simulink model "sm_boom_lift_crawler_test_basket_level_tilt_hydr"  (R2026a)
settings: Solver=ode23t  StopTime=tVec.StopTime  AbsTol=1e-3
PostLoadFcn:
  | sm_boom_lift_crawler_settest('tilt test')
StartFcn:
  | tic;
StopFcn:
  | Elapsed_Sim_Time = toc;
  | %disp(['Elapsed Sim Time = ' num2str(Elapsed_Sim_Time)]);
undefined symbols (not defined in the file): oVec, tVec, X, Y, Z
libraries: sm_boom_lift_crawler_lib x8, nesl_utility x5, sm_lib x3, sm_boom_lift_crawler_lib_actuators x2, sm_boom_lift_crawler_lib_boom x2, fl_lib x2, sm_boom_lift_crawler_lib_inputs x1
Description:
  | Copyright 2025-2026 The MathWorks, Inc.
settings Model: Creator=smiller  LastModifiedBy=smiller
settings SolverCC: MaxConsecutiveMinStep=3
settings DataIOCC: SignalLoggingName=logsout_sm_boom_lift_crawler
settings SimscapeCC: SimscapeNominalValues="[{\"value\":\"1\",\"unit\":\"A\"},{\"value\":\"nomval_psi\",\"unit\":\"psi\"},{\"value\":\"1\",\"unit\":\"cm^2\"},{\"value\":\"nomval_cmv3_s\",\"unit\":\"cm^3/s\"},{\"value\":\"1\",\"unit\":\"kJ/kg\"},{\"value\":\"1\",\"unit\":\"kW\"},{\"value\":\"1\",\"unit\":\"l\"},{\"value\":\"nomval_N\",\"unit\":\"N\"},{\"value\":\"nomval_Nm\",\"unit\":\"N*m\"},{\"value\":\"1\",\"unit\":\"V\"}]"  SimscapeLogName=simlog_sm_boom_lift_crawler  SimscapeLogLimitData=off  SimscapeLogDataHistory=5000.0
settings DiagnosticsConfigSet: SimMechanicsConflictingReferenceFrames=none  SimMechanicsRigidlyBoundBlock=none
settings ExplorerConfigSet: InternalSimMechanicsExplorerSettings="<ExplorerConfiguration><canonicalview>default</canonicalview><AnimationSetting><BasePlaybackSpeed>1.0</BasePlaybackSpeed><PlaybackSpeedFactor>8.0</PlaybackSpeedFactor></AnimationSetting><TilePanel><TileInfo><Tiles Columns=\"1\" Count=\"1\" Rows=\"1\"><Column Weight=\"1\"/><Row Weight=\"1\"/><Tile Height=\"1\" Width=\"1\" X=\"0\" Y=\"0\"/></Tiles></TileInfo><SceneInfo><SceneViewer><BGColor><R>1</R><G>1</G><B>1</B></BGColor><Camera><DoPerspective>on</DoPerspective><Position><X>-2.99999999999999512</X><Y>3.60557049947193109</Y><Z>1.13505049508107825</Z></Position><Center><X>-1.99999999999999512</X><Y>3.60557049947193109</Y><Z>1.13505049508107803</Z></Center><Up><X>0</X><Y>0</Y><Z>1</Z></Up><ViewLimDist>1</ViewLimDist><YLim>0.466307658154998583</YLim><XLim>0.327096812401001136</XLim></Camera></SceneViewer></SceneInfo></TilePanel><MechEditorPanel><Cameras><Camera><Id>Camera8</Id><Value><Name>Extend_Knuckle</Name><NativeCamera><PositionTrackingFeature>Boom.Arms.Telescope.Extend_Cylinder.Transform_Camera_Extend_Knuckle.F</PositionTrackingFeature><CenterTrackingFeature>Boom.Arms.Telescope.Extend_Cylinder.Transform_Camera_Extend_Knuckle.F</CenterTrackingFeature><UpVectorTrackingFeature>Boom.Arms.Telescope.Extend_Cylinder.Transform_Camera_Extend_Knuckle.F</UpVectorTrackingFeature><CenterTrackingOrigin>off</CenterTrackingOrigin><CenterTrackingDirection>-X</CenterTrackingDirection><UpVectorTrackingDirection>-Y</UpVectorTrackingDirection></NativeCamera></Value></Camera><Camera><Id>Camera9</Id><Value><Name>Extend_Basket</Name><NativeCamera><PositionTrackingFeature>Boom.Arms.Telescope.Extend_Cylinder.Transform_Camera_Extend_Basket.F</PositionTrackingFeature><CenterTrackingFeature>Boom.Arms.Telescope.Extend_Cylinder.Transform_Camera_Extend_Basket.F</CenterTrackingFeature><UpVectorTrackingFeature>Boom.Arms.Telescope.Extend_Cylinder.Transform_Camera_Extend_Basket.F</UpVectorTrackingFeature><CenterTrackingOrigin>off</CenterTrackingOrigin><CenterTrackingDirection>+X</CenterTrackingDirection><UpVectorTrackingDirection>+Y</UpVectorTrackingDirection></NativeCamera></Value></Camera><Camera><Id>Camera10</Id><Value><Name>Basket_Rotate</Name><NativeCamera><PositionTrackingFeature>Boom.Basket.Basket_Rotate.Bracket.Reference_Camera_Basket_Rotate_L.R</PositionTrackingFeature><CenterTrackingFeature>Boom.Basket.Basket_Rotate.Bracket.Reference_Camera_Basket_Rotate_L.R</CenterTrackingFeature><UpVectorTrackingFeature>Boom.Basket.Basket_Rotate.Bracket.Reference_Camera_Basket_Rotate_L.R</UpVectorTrackingFeature><CenterTrackingOrigin>off</CenterTrackingOrigin><CenterTrackingDirection>-X</CenterTrackingDirection><UpVectorTrackingDirection>+Z</UpVectorTrackingDirection></NativeCamera></Value></Camera><Camera><Id>Camera11</Id><Value><Name>Tilt_Knuckle</Name><NativeCamera><PositionTrackingFeature>Boom.Arms.Tower.Upper_Knuckle.Reference_Knuckle_Cam.R</PositionTrackingFeature><CenterTrackingFeature>Boom.Arms.Tower.Upper_Knuckle.Reference_Knuckle_Cam.R</CenterTrackingFeature><UpVectorTrackingFeature>Mech_Config.World.W</UpVectorTrackingFeature><CenterTrackingOrigin>off</CenterTrackingOrigin><CenterTrackingDirection>+Z</CenterTrackingDirection><UpVectorTrackingDirection>+Z</UpVectorTrackingDirection></NativeCamera></Value></Camera><Camera><Id>Camera12</Id><Value><Name>Full Test</Name><NativeCamera><PositionKeyframeSet><Keyframe><Time>0</Time><Value><X>-12.242458171438994</X><Y>-0.1433452642095574</Y><Z>4.1505972342390427</Z></Value></Keyframe><Keyframe><Time>69.026826430124729</Time><Value><X>-14.974593328379619</X><Y>0.0056652615564253064</Y><Z>5.3389029552684786</Z></Value></Keyframe><Keyframe><Time>110.29539843687829</Time><Value><X>-21.00761369699504</X><Y>-0.0057417156870510078</Y><Z>8.0689402037867488</Z></Value></Keyframe><Keyframe><Time>140.70430157635164</Time><Value><X>-31.272784439198116</X><Y>-2.5583130214499052e-10</Y><Z>12.723321478963756</Z></Value></Keyframe><Keyframe><Time>181.77628976806102</Time><Value><X>-31.272784439198116</X><Y>-2.5583130214499052e-10</Y><Z>12.723321478963756</Z></Value></Keyframe><Keyframe><Time>208.0087867386398</Time><Value><X>-23.351505250921551</X><Y>-2.5583182919801497e-10</Y><Z>9.1371534281977738</Z></Value></Keyframe><Keyframe><Time>243.06358572448306</Time><Value><X>-16.577121762622586</X><Y>-2.5583144573665537e-10</Y><Z>6.0702143126734844</Z></Value></Keyframe><Keyframe><Time>273.3415757110605</Time><Value><X>-16.577121762622586</X><Y>-2.5583144573665537e-10</Y><Z>6.0702143126734844</Z></Value></Keyframe><Keyframe><Time>321.2447002217541</Time><Value><X>-13.690590902490033</X><Y>0.01787769923724114</Y><Z>4.7891626503614262</Z></Value></Keyframe><Keyframe><Time>350</Time><Value><X>-13.690590902490033</X><Y>0.01787769923724114</Y><Z>4.7891626503614262</Z></Value></Keyframe></PositionKeyframeSet><CenterKeyframeSet><Keyframe><Time>0</Time><Value><X>-4.621228999686064</X><Y>-0.1433452642095574</Y><Z>4.1505972342390436</Z></Value></Keyframe><Keyframe><Time>69.026826430124729</Time><Value><X>-0.17395018713353672</X><Y>0.0056652615564253064</Y><Z>5.3389029552684786</Z></Value></Keyframe><Keyframe><Time>110.29539843687829</Time><Value><X>-9.0038066291239502</X><Y>-0.0057417156870549491</Y><Z>8.0689402037867524</Z></Value></Keyframe><Keyframe><Time>140.70430157635164</Time><Value><X>-14.136391845814327</X><Y>-2.5583979379462107e-10</Y><Z>12.72332147896376</Z></Value></Keyframe><Keyframe><Time>181.77628976806102</Time><Value><X>-2.3429975002054775</X><Y>-2.5584563781180217e-10</Y><Z>12.723321478963761</Z></Value></Keyframe><Keyframe><Time>208.0087867386398</Time><Value><X>-10.17575261115104</X><Y>-2.5583801743778167e-10</Y><Z>9.1371534281977755</Z></Value></Keyframe><Keyframe><Time>243.06358572448306</Time><Value><X>-0.54476849060194255</X><Y>-2.5583897563257738e-10</Y><Z>6.0702143126734844</Z></Value></Keyframe><Keyframe><Time>273.3415757110605</Time><Value><X>-0.11057247639663359</X><Y>-2.5583917956089291e-10</Y><Z>6.0702143126734844</Z></Value></Keyframe><Keyframe><Time>321.2447002217541</Time><Value><X>-5.3452949964231387</X><Y>0.017877699237237366</Y><Z>4.7891626503614253</Z></Value></Keyframe><Keyframe><Time>350</Time><Value><X>-5.3452949964231387</X><Y>0.017877699237237366</Y><Z>4.7891626503614253</Z></Value></Keyframe></CenterKeyframeSet><UpVectorKeyframeSet><Keyframe><Time>0</Time><Value><X>0</X><Y>0</Y><Z>1</Z></Value></Keyframe><Keyframe><Time>69.026826430124729</Time><Value><X>0</X><Y>0</Y><Z>1</Z></Value></Keyframe><Keyframe><Time>110.29539843687829</Time><Value><X>0</X><Y>0</Y><Z>1</Z></Value></Keyframe><Keyframe><Time>140.70430157635164</Time><Value><X>0</X><Y>0</Y><Z>1</Z></Value></Keyframe><Keyframe><Time>181.77628976806102</Time><Value><X>-2.0731981129868445e-16</X><Y>1.0273382740432149e-31</Y><Z>1</Z></Value></Keyframe><Keyframe><Time>208.0087867386398</Time><Value><X>1.4663775813922931e-57</X><Y>2.9591920320379324e-42</Y><Z>1</Z></Value></Keyframe><Keyframe><Time>243.06358572448306</Time><Value><X>1.3898401336634517e-57</X><Y>2.9591920320379324e-42</Y><Z>1</Z></Value></Keyframe><Keyframe><Time>273.3415757110605</Time><Value><X>1.3898401336605064e-57</X><Y>2.9591920320379324e-42</Y><Z>1</Z></Value></Keyframe><Keyframe><Time>321.2447002217541</Time><Value><X>1.3198478700492623e-57</X><Y>2.9591920320379324e-42</Y><Z>1</Z></Value></Keyframe><Keyframe><Time>350</Time><Value><X>1.0642863113510858e-16</X><Y>-4.813997747953607e-32</Y><Z>1</Z></Value></Keyframe></UpVectorKeyframeSet></NativeCamera></Value></Camera><Camera><Id>Camera13</Id><Value><Name>View_Basket_World</Name><NativeCamera><PositionTrackingFeature>Boom.Basket.Basket.Reference_Basket_Cam.R</PositionTrackingFeature><CenterTrackingFeature>Mech_Config.World.W</CenterTrackingFeature><UpVectorTrackingFeature>Boom.Basket.Basket.Reference_Basket_Cam.R</UpVectorTrackingFeature><CenterTrackingOrigin>on</CenterTrackingOrigin><UpVectorTrackingDirection>+Y</UpVectorTrackingDirection></NativeCamera></Value></Camera><Camera><Id>Camera15</Id><Value><Name>Extend_Retract_Pulley</Name><NativeCamera><PositionTrackingFeature>Boom.Arms.Telescope.Extend_Cylinder.Reference_Camera_Retract_Pulley.R</PositionTrackingFeature><CenterTrackingFeature>Boom.Arms.Telescope.Extend_Cylinder.Reference_Camera_Retract_Pulley.R</CenterTrackingFeature><UpVectorTrackingFeature>Boom.Arms.Telescope.Extend_Cylinder.Reference_Camera_Retract_Pulley.R</UpVectorTrackingFeature><CenterTrackingOrigin>off</CenterTrackingOrigin><CenterTrackingDirection>+Y</CenterTrackingDirection><UpVectorTrackingDirection>+Z</UpVectorTrackingDirection></NativeCamera></Value></Camera><Camera><Id>Camera16</Id><Value><Name>Extend_Extend_Pulley</Name><NativeCamera><PositionTrackingFeature>Boom.Arms.Telescope.Extend_Cylinder.Reference_Camera_Extend_Pulley.R</PositionTrackingFeature><CenterTrackingFeature>Boom.Arms.Telescope.Extend_Cylinder.Reference_Camera_Extend_Pulley.R</CenterTrackingFeature><UpVectorTrackingFeature>Boom.Arms.Telescope.Extend_Cylinder.Reference_Camera_Extend_Pulley.R</UpVectorTrackingFeature><CenterTrackingOrigin>off</CenterTrackingOrigin><CenterTrackingDirection>+Z</CenterTrackingDirection><UpVectorTrackingDirection>-Y</UpVectorTrackingDirection></NativeCamera></Value></Camera><Camera><Id>Camera17</Id><Value><Name>Jib</Name><NativeCamera><PositionTrackingFeature>Boom.Basket.Jib.Jib_Mount.Reference_Camera_Basket_Jib.R</PositionTrackingFeature><CenterTrackingFeature>Boom.Basket.Jib.Jib_Mount.Reference_Camera_Basket_Jib.R</CenterTrackingFeature><UpVectorTrackingFeature>Mech_Config.World.W</UpVectorTrackingFeature><CenterTrackingOrigin>off</CenterTrackingOrigin><CenterTrackingDirection>-X</CenterTrackingDirection><UpVectorTrackingDirection>+Z</UpVectorTrackingDirection></NativeCamera></Value></Camera></Cameras><GfxPanelCameraMap><MapElement CameraMLId=\"Camera17\" GfxPanelIndex=\"0\"/></GfxPanelCameraMap><VideoCreator><PlaybackSpeedRatio>8</PlaybackSpeedRatio><FrameRate>30</FrameRate><VideoFormat>MPEG-4</VideoFormat><FrameSize>auto</FrameSize></VideoCreator></MechEditorPanel></ExplorerConfiguration>"

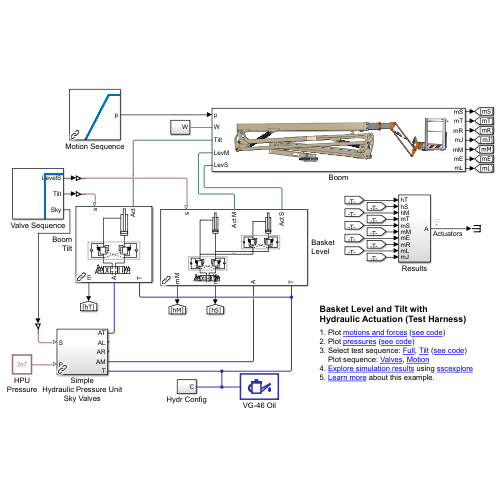
[thumbnail: Simulink's stored preview of the top-level diagram]
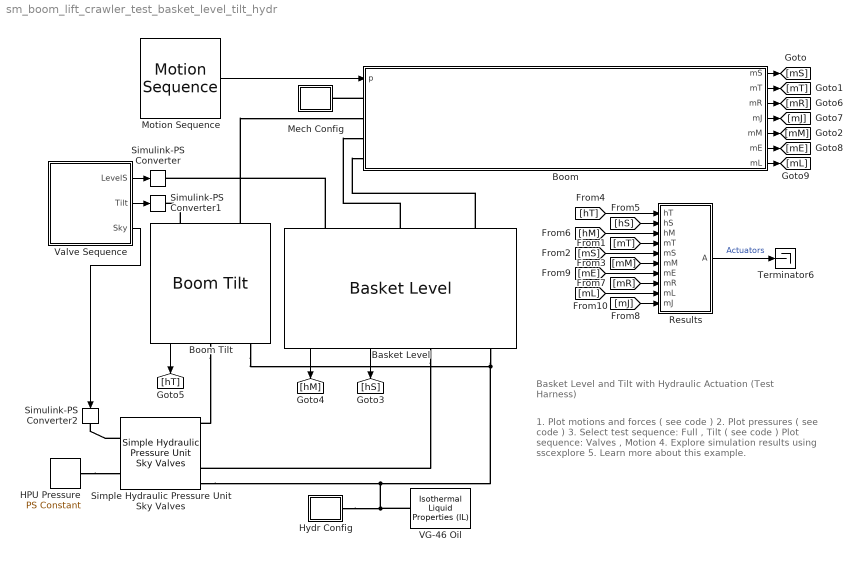
== system sm_boom_lift_crawler_test_basket_level_tilt_hydr ==
  note: Basket Level and Tilt with
      | Hydraulic Actuation (Test Harness)
  note: 1. Plot motions and forces ( see code )
      | 2. Plot pressures ( see code )
      | 3. Select test sequence: Full , Tilt ( see code )
      | Plot sequence: Valves , Motion
      | 4. Explore simulation results using sscexplore
      | 5. Learn more about this example.
  Basket Level : sm_boom_lift_crawler_lib_actuators/Actuators/Sky Manifold/Sky Valves II/Basket Level  SystemSampleTime=-1  VariantActivationTime=update diagram  EmptyChoice=off  PassThrough=off  PassThroughVariantControl=(default)  EmptyChoiceVariantControl=(default)  AllowFlexibleInterface=on  Latency=0  AutoFrameSizeCalculation=off
  Boom : Subsystem
      mask Display: image('sm002.svg');
  Boom Tilt : sm_boom_lift_crawler_lib_actuators/Actuators/Sky Manifold/Sky Valves I/Boom Tilt  SystemSampleTime=-1  VariantActivationTime=update diagram  EmptyChoice=off  PassThrough=off  PassThroughVariantControl=(default)  EmptyChoiceVariantControl=(default)  AllowFlexibleInterface=on  Latency=0  AutoFrameSizeCalculation=off
  HPU Pressure : fl_lib/Physical Signals/Sources/PS Constant  constant=2e7 Pa
  Hydr Config : Subsystem
  Mech Config : Subsystem
  Motion Sequence : sm_boom_lift_crawler_lib_inputs/Motion Sequence  SystemSampleTime=-1  VariantActivationTime=update diagram  EmptyChoice=off  PassThrough=off  PassThroughVariantControl=(default)  EmptyChoiceVariantControl=(default)  AllowFlexibleInterface=on  Latency=0  AutoFrameSizeCalculation=off
  Results : Subsystem
  Simple Hydraulic Pressure Unit Sky Valves : sm_boom_lift_crawler_lib/Simple Hydraulic Pressure Unit Sky Valves  SystemSampleTime=-1  VariantActivationTime=update diagram  EmptyChoice=off  PassThrough=off  PassThroughVariantControl=(default)  EmptyChoiceVariantControl=(default)  AllowFlexibleInterface=on  Latency=0  AutoFrameSizeCalculation=off
  Simulink-PS Converter : nesl_utility/Simulink-PS Converter  PhysicalDomain=network_engine_domain  SubClassName=ps_input  LeftPortType=input  RightPortType=output  PseudoPeriodic=off  Frequencies=[]  NoiseDistribution=none  NoiseParameters=[]  Unit=1  AffineConversion=off  FilteringAndDerivatives=provide  SimscapeFilterOrder=1  InputFilterTimeConstant=0.001  UdotUserProvided=0
  Simulink-PS Converter1 : nesl_utility/Simulink-PS Converter  PhysicalDomain=network_engine_domain  SubClassName=ps_input  LeftPortType=input  RightPortType=output  PseudoPeriodic=off  Frequencies=[]  NoiseDistribution=none  NoiseParameters=[]  Unit=1  AffineConversion=off  FilteringAndDerivatives=provide  SimscapeFilterOrder=1  InputFilterTimeConstant=0.001  UdotUserProvided=0
  Simulink-PS Converter2 : nesl_utility/Simulink-PS Converter  PhysicalDomain=network_engine_domain  SubClassName=ps_input  LeftPortType=input  RightPortType=output  PseudoPeriodic=off  Frequencies=[]  NoiseDistribution=none  NoiseParameters=[]  Unit=1  AffineConversion=off  FilteringAndDerivatives=provide  SimscapeFilterOrder=1  InputFilterTimeConstant=0.001  UdotUserProvided=0
  Terminator6 : Terminator
  VG-46 Oil : fl_lib/Isothermal Liquid/Utilities/Isothermal Liquid Properties (IL)  rho_L_atm=867.346 kg/m^3  bulk_modulus_model=foundation.enum.bulk_modulus_model.const  beta_gain=6  beta_L_atm=1.48150e+09 Pa  nu_atm=(45.7333)*(1) cSt  p_atm=0.101325 MPa  p_min=1 Pa  properties_range_check=simscape.enum.assert.action.error  air_fraction=ratio_dissolved_air  polytropic_index=1.0  rho_g_atm=1.225 kg/m^3  air_dissolution_model=simscape.enum.onoff.off  p_crit=3 MPa
  Valve Sequence : Subsystem
      mask Display: image('sm_boom_lift_crawler_valve_seq_outputonly.svg');
  wires:
  Boom/7(mL) -> [mL]
  Boom/4(mJ) -> [mJ]
  Boom/1(mS) -> [mS]
  Valve Sequence/2(Tilt) -> Simulink-PS Converter1/1
  Boom Tilt/1 -> [hT]
  Boom/5(mM) -> [mM]
  [hT] -> Results/1(hT)
  Results/1(A) -> Terminator6/1  "Actuators"
  Valve Sequence/1(LevelS) -> Simulink-PS Converter/1
  Basket Level/2 -> [hS]
  Boom/6(mE) -> [mE]
  Valve Sequence/3(Sky) -> Simulink-PS Converter2/1
  Boom/2(mT) -> [mT]
  [mE] -> Results/7(mE)
  Basket Level/1 -> [hM]
  Boom/3(mR) -> [mR]
  [mR] -> Results/8(mR)
  [mJ] -> Results/10(mJ)
  [mM] -> Results/6(mM)
  [mS] -> Results/5(mS)
  [mT] -> Results/4(mT)
  [mL] -> Results/9(mL)
  [hM] -> Results/3(hM)
  Motion Sequence/1 -> Boom/1(p)
  [hS] -> Results/2(hS)
  connections:
  Boom Tilt/RConn2 -- VG-46 Oil/RConn1 -- Hydr Config/RConn1 -- Simple Hydraulic Pressure Unit Sky Valves/RConn5 -- Basket Level/RConn2
  Boom Tilt/RConn1 -- Simple Hydraulic Pressure Unit Sky Valves/RConn1
  Basket Level/RConn1 -- Simple Hydraulic Pressure Unit Sky Valves/RConn4
  Simple Hydraulic Pressure Unit Sky Valves/LConn1 -- Simulink-PS Converter2/RConn1
  Basket Level/LConn2 -- Boom/LConn3
  Boom Tilt/LConn1 -- Simulink-PS Converter1/RConn1
  HPU Pressure/RConn1 -- Simple Hydraulic Pressure Unit Sky Valves/LConn2
  Boom Tilt/LConn2 -- Boom/LConn2
  Basket Level/LConn3 -- Boom/LConn4
  Boom/LConn1 -- Mech Config/LConn1
  Basket Level/LConn1 -- Simulink-PS Converter/RConn1

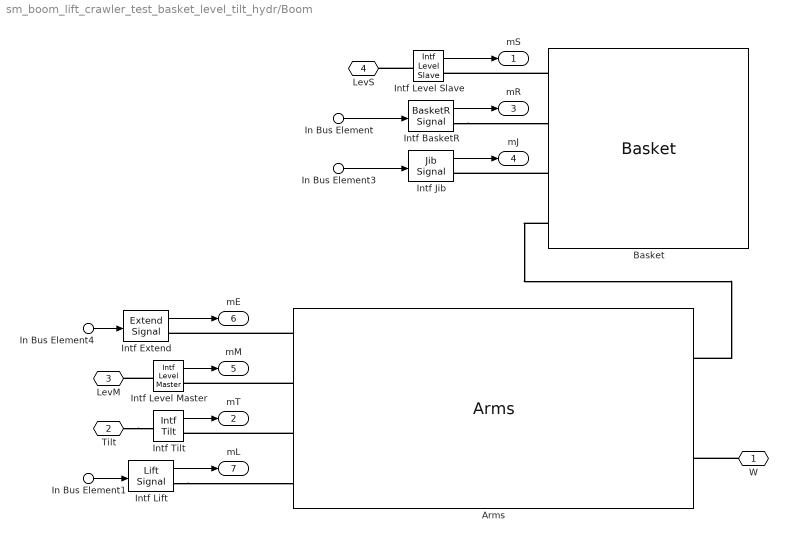
== system sm_boom_lift_crawler_test_basket_level_tilt_hydr/Boom ==
  In Bus Element : Inport  PortName=p  Element=BasketR
  In Bus Element3 : Inport  PortName=p  Element=Jib
  In Bus Element4 : Inport  PortName=p  Element=Extend
  In Bus Element1 : Inport  PortName=p  Element=Lift
  Arms : sm_boom_lift_crawler_lib_boom/Boom/Arms  SystemSampleTime=-1  VariantActivationTime=update diagram  EmptyChoice=off  PassThrough=off  PassThroughVariantControl=(default)  EmptyChoiceVariantControl=(default)  AllowFlexibleInterface=on  Latency=0  AutoFrameSizeCalculation=off
  Basket : sm_boom_lift_crawler_lib_boom/Boom/Basket  SystemSampleTime=-1  VariantActivationTime=update diagram  EmptyChoice=off  PassThrough=off  PassThroughVariantControl=(default)  EmptyChoiceVariantControl=(default)  AllowFlexibleInterface=on  Latency=0  AutoFrameSizeCalculation=off
  Intf BasketR : sm_boom_lift_crawler_lib/BasketR Signal  SystemSampleTime=-1  VariantActivationTime=update diagram  EmptyChoice=off  PassThrough=off  PassThroughVariantControl=(default)  EmptyChoiceVariantControl=(default)  AllowFlexibleInterface=on  Latency=0  AutoFrameSizeCalculation=off
  Intf Extend : sm_boom_lift_crawler_lib/Extend Signal  SystemSampleTime=-1  VariantActivationTime=update diagram  EmptyChoice=off  PassThrough=off  PassThroughVariantControl=(default)  EmptyChoiceVariantControl=(default)  AllowFlexibleInterface=on  Latency=0  AutoFrameSizeCalculation=off
  Intf Jib : sm_boom_lift_crawler_lib/Jib Signal  SystemSampleTime=-1  VariantActivationTime=update diagram  EmptyChoice=off  PassThrough=off  PassThroughVariantControl=(default)  EmptyChoiceVariantControl=(default)  AllowFlexibleInterface=on  Latency=0  AutoFrameSizeCalculation=off
  Intf Level Master : sm_boom_lift_crawler_lib/Intf Level Master  SystemSampleTime=-1  VariantActivationTime=update diagram  EmptyChoice=off  PassThrough=off  PassThroughVariantControl=(default)  EmptyChoiceVariantControl=(default)  AllowFlexibleInterface=on  Latency=0  AutoFrameSizeCalculation=off
  Intf Level Slave : sm_boom_lift_crawler_lib/Intf Level Slave  SystemSampleTime=-1  VariantActivationTime=update diagram  EmptyChoice=off  PassThrough=off  PassThroughVariantControl=(default)  EmptyChoiceVariantControl=(default)  AllowFlexibleInterface=on  Latency=0  AutoFrameSizeCalculation=off
  Intf Lift : sm_boom_lift_crawler_lib/Lift Signal  SystemSampleTime=-1  VariantActivationTime=update diagram  EmptyChoice=off  PassThrough=off  PassThroughVariantControl=(default)  EmptyChoiceVariantControl=(default)  AllowFlexibleInterface=on  Latency=0  AutoFrameSizeCalculation=off
  Intf Tilt : sm_boom_lift_crawler_lib/Intf Tilt  SystemSampleTime=-1  VariantActivationTime=update diagram  EmptyChoice=off  PassThrough=off  PassThroughVariantControl=(default)  EmptyChoiceVariantControl=(default)  AllowFlexibleInterface=on  Latency=0  AutoFrameSizeCalculation=off
  W : PMIOPort  Side=Left
  Tilt : PMIOPort  Port=2  Side=Left
  LevM : PMIOPort  Port=3  Side=Left
  LevS : PMIOPort  Port=4  Side=Left
  mS : Outport
  mT : Outport  Port=2
  mR : Outport  Port=3
  mJ : Outport  Port=4
  mM : Outport  Port=5
  mE : Outport  Port=6
  mL : Outport  Port=7
  wires:
  Intf Level Slave/1 -> mS/1
  Intf Tilt/1 -> mT/1
  Intf Level Master/1 -> mM/1
  Intf BasketR/1 -> mR/1
  In Bus Element/1 -> Intf BasketR/1
  In Bus Element3/1 -> Intf Jib/1
  Intf Jib/1 -> mJ/1
  In Bus Element4/1 -> Intf Extend/1
  Intf Extend/1 -> mE/1
  Intf Lift/1 -> mL/1
  In Bus Element1/1 -> Intf Lift/1
  connections:
  Basket/RConn3 -- Intf Jib/RConn1
  Arms/LConn3 -- Intf Tilt/RConn1
  Basket/RConn4 -- Arms/RConn1
  Intf BasketR/RConn1 -- Basket/RConn2
  Basket/RConn1 -- Intf Level Slave/RConn1
  Intf Level Master/LConn1 -- LevM/RConn1
  Arms/LConn2 -- Intf Level Master/RConn1
  W/RConn1 -- Arms/RConn2
  Intf Level Slave/LConn1 -- LevS/RConn1
  Tilt/RConn1 -- Intf Tilt/LConn1
  Arms/LConn1 -- Intf Extend/RConn1
  Intf Lift/RConn1 -- Arms/LConn4

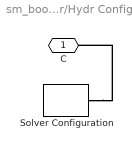
== system sm_boom_lift_crawler_test_basket_level_tilt_hydr/Hydr Config ==
  Solver Configuration : nesl_utility/Solver Configuration  PhysicalDomain=network_engine_domain  SubClassName=solver  LeftPortType=input  RightPortType=generic  Tones=[]  Harmonics=[]  SimulateNoise=off  Profile=off  UseLocalSampling=off  EnableSwitchedLinearOptims=on  FrequencyDomain=off  UseCCode=off  RelTol=0.001  AbsTol=1e-06  MinStep=1e-09  ToWorkspace=off  RevertToSquareIcSolve=off  NumHomotopyIterations=100  PhasorMode=off  PhasorModeNumHarmonics=1  ConsistencySolver=NEWTON_FTOL  CanonicalOrdering=UNORDERED  OptimizeIntermediates=UNOPTIMIZED  IndexReductionMethod=DerivativeReplacement  DoDC=off  ResidualTolerance=1e-9  ConsistencyTolSource=GLOBAL  ConsistencyAbsTol=0.001  ConsistencyRelTol=0.001  ConsistencyTolFactor=0.001  UseLocalSolver=off  LocalSolverChoice=NE_BACKWARD_EULER_ADVANCER  ResolveIndetEquations=on  FunctionEvalNumThread=1  LocalSolverSampleTime=2e-3  DoFixedCost=off  MaxNonlinIter=5  MaxModeIter=2  ComputeImpulses=off  ImpulseIterations=2  LinearAlgebra=Sparse  LinearAlgebraNumThread=0  EquationFormulation=NE_TIME_EF  DelaysMemoryBudget=1024  AutomaticFiltering=on  FilteringTimeConstant=1e-3  PartitionStorageMethod=EXHAUSTIVE  PartitionMemoryBudget=1024  PartitionMethod=FAST  MultibodyUseLocalSolver=off  MultibodyLocalSolverChoice=ODE1  MultibodyLocalSolverSampleTime=0.001
  C : PMIOPort  Side=Right
  connections:
  Solver Configuration/RConn1 -- C/RConn1

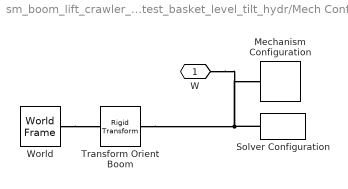
== system sm_boom_lift_crawler_test_basket_level_tilt_hydr/Mech Config ==
  Mechanism Configuration : sm_lib/Utilities/Mechanism Configuration  UniformGravity=Constant  GravityVector=[0 0 -9.80665]  GravityVectorUnits=m/s^2  LinearizationDelta=0.001  JointModeTransitionNonlinearIterations=2
  Solver Configuration : nesl_utility/Solver Configuration  PhysicalDomain=network_engine_domain  SubClassName=solver  LeftPortType=input  RightPortType=generic  Tones=[]  Harmonics=[]  SimulateNoise=off  Profile=off  UseLocalSampling=off  EnableSwitchedLinearOptims=on  FrequencyDomain=off  UseCCode=off  RelTol=0.001  AbsTol=1e-06  MinStep=1e-09  ToWorkspace=off  RevertToSquareIcSolve=off  NumHomotopyIterations=100  PhasorMode=off  PhasorModeNumHarmonics=1  ConsistencySolver=NEWTON_FTOL  CanonicalOrdering=UNORDERED  OptimizeIntermediates=UNOPTIMIZED  IndexReductionMethod=DerivativeReplacement  DoDC=off  ResidualTolerance=1e-9  ConsistencyTolSource=GLOBAL  ConsistencyAbsTol=0.001  ConsistencyRelTol=0.001  ConsistencyTolFactor=0.001  UseLocalSolver=off  LocalSolverChoice=NE_BACKWARD_EULER_ADVANCER  ResolveIndetEquations=on  FunctionEvalNumThread=1  LocalSolverSampleTime=2e-3  DoFixedCost=off  MaxNonlinIter=3  MaxModeIter=2  ComputeImpulses=off  ImpulseIterations=2  LinearAlgebra=auto  LinearAlgebraNumThread=0  EquationFormulation=NE_TIME_EF  DelaysMemoryBudget=1024  AutomaticFiltering=on  FilteringTimeConstant=0.001  PartitionStorageMethod=AS_NEEDED  PartitionMemoryBudget=1024  PartitionMethod=ROBUST  MultibodyUseLocalSolver=off  MultibodyLocalSolverChoice=ODE1  MultibodyLocalSolverSampleTime=0.001
  Transform Orient Boom : sm_lib/Frames and Transforms/Rigid Transform  RotationMethod=StandardAxis  FollAlignAxisA=+X  BaseAlignAxisA=+Y  FollAlignAxisB=+Y  BaseAlignAxisB=+Z  RotationStandardAxis=+Z  RotationAngle=180  RotationAngleUnits=deg  RotationArbitraryAxis=[0 0 1]  RotationSequenceAxes=FollowerAxes  RotationSequence=XYX  RotationSequenceAngles=[0 0 0]  RotationSequenceAnglesUnits=deg  RotationMatrix=[1 0 0; 0 1 0; 0 0 1]  Quaternion=[1 0 0 0]  TranslationMethod=None  TranslationCartesianOffset=[0 0 0]  TranslationCartesianOffsetUnits=m  TranslationStandardAxis=+Z  TranslationStandardOffset=0  TranslationStandardOffsetUnits=m  TranslationROffset=0  TranslationROffsetUnits=m  TranslationThetaOffset=0  TranslationThetaOffsetUnits=deg  TranslationZOffset=0  TranslationZOffsetUnits=m
  World : sm_lib/Frames and Transforms/World Frame
  W : PMIOPort  Side=Left
  connections:
  Solver Configuration/RConn1 -- Transform Orient Boom/RConn1 -- W/RConn1 -- Mechanism Configuration/RConn1
  World/RConn1 -- Transform Orient Boom/LConn1

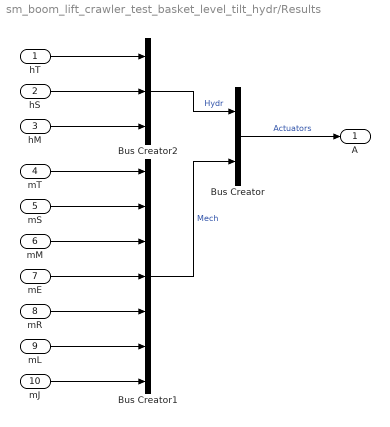
== system sm_boom_lift_crawler_test_basket_level_tilt_hydr/Results ==
  hT : Inport
  hS : Inport  Port=2
  hM : Inport  Port=3
  mT : Inport  Port=4
  mS : Inport  Port=5
  mM : Inport  Port=6
  mE : Inport  Port=7
  mR : Inport  Port=8
  mL : Inport  Port=9
  mJ : Inport  Port=10
  Bus Creator : BusCreator  Inputs=2
  Bus Creator1 : BusCreator  Inputs=7
  Bus Creator2 : BusCreator  Inputs=3
  A : Outport
  wires:
  hT/1 -> Bus Creator2/1
  Bus Creator/1 -> A/1  "Actuators"
  Bus Creator1/1 -> Bus Creator/2  "Mech"
  Bus Creator2/1 -> Bus Creator/1  "Hydr"
  mT/1 -> Bus Creator1/1
  mS/1 -> Bus Creator1/2
  mM/1 -> Bus Creator1/3
  hS/1 -> Bus Creator2/2
  hM/1 -> Bus Creator2/3
  mE/1 -> Bus Creator1/4
  mR/1 -> Bus Creator1/5
  mL/1 -> Bus Creator1/6
  mJ/1 -> Bus Creator1/7

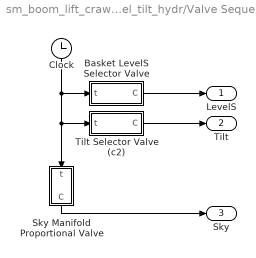
== system sm_boom_lift_crawler_test_basket_level_tilt_hydr/Valve Sequence ==
  Basket LevelS Selector Valve : Subsystem
  Clock : Clock
  Sky Manifold Proportional Valve : Subsystem
  Tilt Selector Valve (c2) : Subsystem
  LevelS : Outport
  Tilt : Outport  Port=2
  Sky : Outport  Port=3
  wires:
  Basket LevelS Selector Valve/1(C) -> LevelS/1
  Clock/1 -> Sky Manifold Proportional Valve/1(t), Tilt Selector Valve (c2)/1(t), Basket LevelS Selector Valve/1(t)
  Sky Manifold Proportional Valve/1(C) -> Sky/1
  Tilt Selector Valve (c2)/1(C) -> Tilt/1

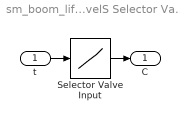
== system sm_boom_lift_crawler_test_basket_level_tilt_hydr/Valve Sequence/Basket LevelS Selector Valve ==
  t : Inport
  Selector Valve Input : Lookup_n-D  NumberOfTableDimensions=1  BreakpointsForDimension1=[0 1]  Table=[0 0]  InterpMethod=Flat  ExtrapMethod=Clip  UseLastTableValue=on  InternalRulePriority=Speed  RndMeth=Simplest
  C : Outport
  wires:
  t/1 -> Selector Valve Input/1
  Selector Valve Input/1 -> C/1

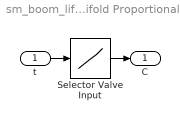
== system sm_boom_lift_crawler_test_basket_level_tilt_hydr/Valve Sequence/Sky Manifold Proportional Valve ==
  t : Inport
  Selector Valve Input : Lookup_n-D  NumberOfTableDimensions=1  BreakpointsForDimension1=tVec.sky.proportional  Table=oVec.sky.proportional  InterpMethod=Flat  ExtrapMethod=Clip  UseLastTableValue=on  InternalRulePriority=Speed  RndMeth=Simplest
  C : Outport
  wires:
  t/1 -> Selector Valve Input/1
  Selector Valve Input/1 -> C/1

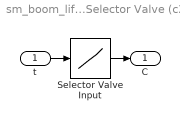
== system sm_boom_lift_crawler_test_basket_level_tilt_hydr/Valve Sequence/Tilt Selector Valve (c2) ==
  t : Inport
  Selector Valve Input : Lookup_n-D  NumberOfTableDimensions=1  BreakpointsForDimension1=tVec.sky.c2.all  Table=oVec.sky.c2.all  InterpMethod=Flat  ExtrapMethod=Clip  UseLastTableValue=on  InternalRulePriority=Speed  RndMeth=Simplest
  C : Outport
  wires:
  Selector Valve Input/1 -> C/1
  t/1 -> Selector Valve Input/1
